simulink model "ACC_QP"  (R2024b)
settings: Solver=ode15s  StartTime=0.0  StopTime=100  RelTol=1e-3
values from neighbouring files (symbols this model uses):
  M = 1650    [File.mat]
  rk = block.InputPort(3).Data    [Data_driven_CLF_CBF_QP.m]    (also in File.mat = 25)
  T = 0.1    [File.mat]
  x0 = [81 17]    [File.mat]
libraries: autolibshared x1
settings Model: SetupFcn=setupFcn  SimulationMode=accelerator  Creator=12775  LastModifiedBy=12775
settings ModelReferenceCC: EnableRefExpFcnMdlSchedulingChecks=on  EnableParallelModelReferenceBuilds=on  ParallelModelReferenceMATLABWorkerInit=Load Top Model  SupportModelReferenceSimTargetCustomCode=on

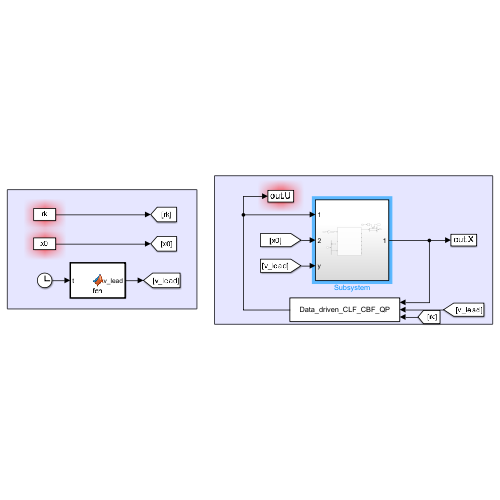
[thumbnail: Simulink's stored preview of the top-level diagram]
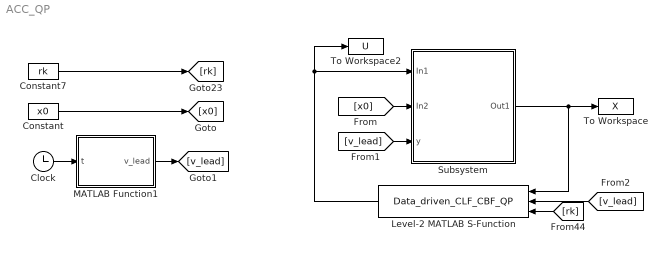
== system ACC_QP ==
  Clock : Clock
  Constant : Constant  Value=x0
  Constant7 : Constant  Value=rk
  Level-2 MATLAB S-Function : M-S-Function  FunctionName=Data_driven_CLF_CBF_QP  Parameters=Params
  MATLAB Function1 : MATLAB Function  TreatAsAtomicUnit=on
  Subsystem : Subsystem
  To Workspace : ToWorkspace  VariableName=X  SaveFormat=Structure With Time  SampleTime=-1
  To Workspace2 : ToWorkspace  VariableName=U  SaveFormat=Structure With Time  SampleTime=T
  wires:
  Subsystem/1(Out1) -> Level-2 MATLAB S-Function/1, To Workspace/1
  Clock/1 -> MATLAB Function1/1(t)
  Constant/1 -> [x0]
  MATLAB Function1/1(v_lead) -> [v_lead]
  [x0] -> Subsystem/2(In2)
  [v_lead] -> Subsystem/3(y)
  [v_lead] -> Level-2 MATLAB S-Function/2
  Constant7/1 -> [rk]
  [rk] -> Level-2 MATLAB S-Function/3
  Level-2 MATLAB S-Function/1 -> To Workspace2/1, Subsystem/1(In1)

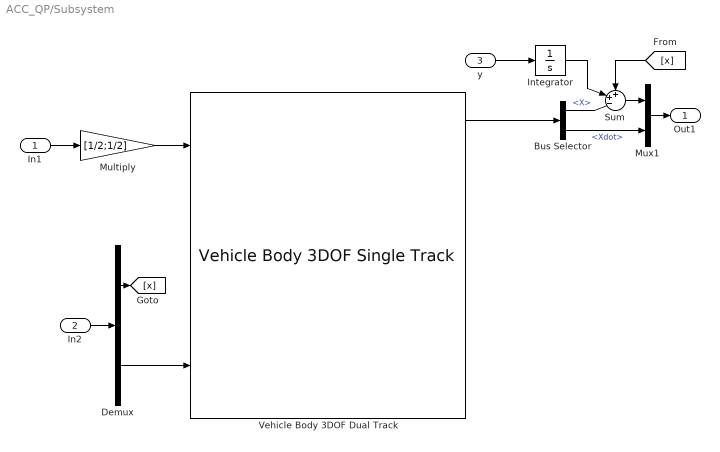
== system ACC_QP/Subsystem ==
  In1 : Inport
  In2 : Inport  Port=2
  y : Inport  Port=3
  Bus Selector : BusSelector  OutputSignals=InertFrm.Cg.Disp.X,InertFrm.Cg.Vel.Xdot
  Demux : Demux  Outputs=2
  Integrator : Integrator
  Multiply : Gain  Gain=[1/2;1/2]
  Mux1 : Mux  Inputs=2
  Sum : Sum  Inputs=++-|
  Vehicle Body 3DOF Dual Track : autolibshared/Vehicle Body 3DOF Single Track  trackMode=Dual  inputMode=External longitudinal forces  frontSteerMode=off  rearSteerMode=off  windMode=off  muMode=off  extFMode=off  extMMode=off  htchFMode=off  htchMMode=off  extXo=off  extpsio=off  extxdoto=on  extro=off  extYo=off  extTamb=off  extydoto=off  aMode=2  NF=2  NR=2  m=M  a=1.4  b=1.6  h=0.35  dh=1  hh=0.2  X_o=0  xdot_o=0  CalphaMode=off  sigmaMode=off  d=0  hl=0  w=[1.4,1.4]  Cy_f=12e3  Cy_r=11e3  sigma_f=.1  sigma_r=.1  alpha_f_brk=[-.1 .1]  Cy_f_data=[-9e3 9e3]  alpha_r_brk=[-.1 .1]  Cy_r_data=[-9e3 9e3]  Y_o=0  ydot_o=0  Izz=4000  psi_o=0  r_o=0  Af=2  Cd=.3  Cl=.1  Cpm=.1  beta_w=[0 0.01:0.01:0.3]  Cs=[0:0.03:0.9]  Cym=[0 1e-6:0.01:0.3]  Pabs=101325  Tair=273  g=9.81  mu=1  xdot_tol=.01  Fznom=5000  Fxtire_sat=7e4  Fytire_sat=7e4  longOff=0  latOff=0  vertOff=0  wrapAng=off
      settings: LibrarySourceBlock=vehdynlibeom/Vehicle Body 3DOF Dual Track
  Out1 : Outport
  wires:
  In2/1 -> Demux/1
  Multiply/1 -> Vehicle Body 3DOF Dual Track/1
  Bus Selector/2 -> Mux1/2  "<Xdot>"
  Mux1/1 -> Out1/1
  Vehicle Body 3DOF Dual Track/1 -> Bus Selector/1
  Demux/2 -> Vehicle Body 3DOF Dual Track/3
  Demux/1 -> [x]
  y/1 -> Integrator/1
  Sum/1 -> Mux1/1
  Bus Selector/1 -> Sum/3  "<X>"
  In1/1 -> Multiply/1
  [x] -> Sum/1
  Integrator/1 -> Sum/2

== matlab function ACC_QP/MATLAB Function1 ==
  data: t input; v_lead output
function v_lead = fcn(t)
    t_points = [0, 10, 20, 30, 40, 50, 60, 100];
    v_points = [16, 16, 22.5, 22.5, 25, 25,16, 16];
    
    % 根据输入时间t找到对应的速度值
    v_lead = 16; % 默认值
    for i = 1:length(t_points) - 1
        if t >= t_points(i) && t <= t_points(i + 1)
            % 插值计算
            v_lead = v_points(i) + ((v_points(i + 1) - v_points(i)) / (t_points(i + 1) - t_points(i))) * (t - t_points(i));
            break;
        end
    end
end
